simulink model "mixTest123"  (R2020a)
settings: Solver=VariableStepAuto  StartTime=0.0  StopTime=1000  FixedStep=0.05  RelTol=1e-3
InitFcn:
  | data_current
values from neighbouring files (symbols this model uses):
  a1 = rho * D^4 * alpha1    (= 0.000388302366464)    [data_current.m]    (also in main_init.m)
  a2 = -rho * D^3 * alpha2 * (1 - omega)    (= 0.0037030698432)    [data_current.m]    (also in main_init.m)
  ag = [Ax Ay Az]'    [init_modello.m]
  alpha1 = 0.0113    [data_current.m]    (also in main_init.m)
  alpha2 = -0.0091    [data_current.m]    (also in main_init.m)
  areaOfInterestCorner = [42.317744;10.915136; 0]    [init_controllo.m]    (also in missionA.m = [42.317744)
  bg = [Bx By Bz]'    [init_modello.m]
  cd_pitch = 0.7    [init_modello.m]
  cd_roll = 0.04    [init_modello.m]
  cd_x = 0.4    [init_modello.m]
  cd_y = 1    [init_modello.m]
  cd_yaw = 0.7    [init_modello.m]
  cd_z = 1    [init_modello.m]
  cg = [Cx Cy Cz]'    [init_modello.m]
  D = 0.076    [data_current.m]    (also in main_init.m)
  dead_zone_limit = 31.5    [data_current.m]    (also in main_init.m)
  dg = [Dx Dy Dz]'    [init_modello.m]
  eg = [Ex Ey Ez]'    [init_modello.m]
  fg = [Fx Fy Fz]'    [init_modello.m]
  g = 9.81    [init_modello.m]
  galleggiamento = 66.5386    [init_controllo.m]
  gg = [Gx Gy Gz]'    [init_modello.m]
  H0 = 0    [init_modello.m]
  init_position = [pointP(1),pointP(2),0.15,0,0,deg2rad(angle)]'    [appunti.m]    (also in init_modello.m = [pointP(1),pointP(2),0.15,0,0,deg2rad(alpha)]')
  init_velocity = [0 0 0 0 0 0]'    [init_modello.m]
  Ixx = 0.93304097392    [init_modello.m]
  Ixy = 0    [init_modello.m]
  Ixz = 0    [init_modello.m]
  Iyy = 25.58745481378    (= 25.5874548138)    [init_modello.m]
  Iyz = 0    [init_modello.m]
  Izz = 25.58745481378    (= 25.5874548138)    [init_modello.m]
  K_i_heave_div = 20    [init_controllo.m]
  K_i_heave_pos = 1    [init_controllo.m]
  K_i_heave_surf = 20    [init_controllo.m]
  K_i_heave_trans = 5    [init_controllo.m]
  K_i_heave_turn = 5    [init_controllo.m]
  K_i_pitch_div = 0    [init_controllo.m]
  K_i_pitch_pos = 0.1*0    (= 0)    [init_controllo.m]
  K_i_pitch_surf = 0    [init_controllo.m]
  K_i_pitch_trans = 0    [init_controllo.m]
  K_i_pitch_turn = 0    [init_controllo.m]
  K_i_roll_div = 0    [init_controllo.m]
  K_i_roll_pos = 0.1*0    (= 0)    [init_controllo.m]
  K_i_roll_surf = 1    [init_controllo.m]
  K_i_roll_trans = 0    [init_controllo.m]
  K_i_roll_turn = 0    [init_controllo.m]
  K_i_surge_div = 3    [init_controllo.m]
  K_i_surge_pos = 0.1679*30    (= 5.037)    [init_controllo.m]
  K_i_surge_surf = 3    [init_controllo.m]
  K_i_surge_trans = 0.1679*15    (= 2.5185)    [init_controllo.m]
  K_i_surge_turn = 0.1679*60    (= 10.074)    [init_controllo.m]
  K_i_sway_div = 6    [init_controllo.m]
  K_i_sway_pos = 5    [init_controllo.m]
  K_i_sway_surf = 3    [init_controllo.m]
  K_i_sway_trans = 2    [init_controllo.m]
  K_i_sway_turn = 50    [init_controllo.m]
  K_i_yaw_div = 0    [init_controllo.m]
  K_i_yaw_pos = 1    [init_controllo.m]
  K_i_yaw_surf = 0    [init_controllo.m]
  K_i_yaw_trans = 20    [init_controllo.m]
  K_i_yaw_turn = 3    [init_controllo.m]
  K_p_heave_div = 200    [init_controllo.m]
  K_p_heave_pos = 320    [init_controllo.m]
  K_p_heave_surf = 200    [init_controllo.m]
  K_p_heave_trans = 170    [init_controllo.m]
  K_p_heave_turn = 170    [init_controllo.m]
  K_p_phi_div = 0.15    [init_controllo.m]
  K_p_phi_pos = 1*0.1    (= 0.1)    [init_controllo.m]
  K_p_phi_surf = 0.15    [init_controllo.m]
  K_p_phi_trans = 0.1    [init_controllo.m]
  K_p_phi_turn = 0.1    [init_controllo.m]
  K_p_pitch_div = 50    [init_controllo.m]
  K_p_pitch_pos = 25    [init_controllo.m]
  K_p_pitch_surf = 50    [init_controllo.m]
  K_p_pitch_trans = 25    [init_controllo.m]
  K_p_pitch_turn = 25    [init_controllo.m]
  K_p_psi_div = 0.3    [init_controllo.m]
  K_p_psi_pos = 0.25    [init_controllo.m]
  K_p_psi_surf = 0.3    [init_controllo.m]
  K_p_psi_trans = 0.2    [init_controllo.m]
  K_p_roll_div = 10    [init_controllo.m]
  K_p_roll_pos = 0.1*40    (= 4)    [init_controllo.m]
  K_p_roll_surf = 10    [init_controllo.m]
  K_p_roll_trans = 0.1*40    (= 4)    [init_controllo.m]
  K_p_roll_turn = 4    [init_controllo.m]
  K_p_surge_div = 80    [init_controllo.m]
  K_p_surge_pos = 13.7782*2.5    (= 34.4455)    [init_controllo.m]
  K_p_surge_surf = 80    [init_controllo.m]
  K_p_surge_trans = 20    [init_controllo.m]
  K_p_surge_turn = 150    [init_controllo.m]
  K_p_sway_div = 100    [init_controllo.m]
  K_p_sway_pos = 90    [init_controllo.m]
  K_p_sway_surf = 80    [init_controllo.m]
  K_p_sway_trans = 80    [init_controllo.m]
  K_p_sway_turn = 200    [init_controllo.m]
  K_p_th_div = 0.3    [init_controllo.m]
  K_p_th_pos = 0.1    [init_controllo.m]
  K_p_th_surf = 0.3    [init_controllo.m]
  K_p_th_trans = 0.1    [init_controllo.m]
  K_p_th_turn = 0.1    [init_controllo.m]
  K_p_x_div = 0.12    [init_controllo.m]
  K_p_x_pos = 0.12    [init_controllo.m]
  K_p_x_surf = 0.12    [init_controllo.m]
  K_p_y_div = 0.6    [init_controllo.m]
  K_p_y_pos = 0.34    [init_controllo.m]
  K_p_y_surf = 0.1    [init_controllo.m]
  K_p_y_trans = 0.3    [init_controllo.m]
  K_p_y_turn = 0.3    [init_controllo.m]
  K_p_yaw_div = 70    [init_controllo.m]
  K_p_yaw_pos = 20    [init_controllo.m]
  K_p_yaw_surf = 70    [init_controllo.m]
  K_p_yaw_trans = 160    [init_controllo.m]
  K_p_yaw_turn = 60    [init_controllo.m]
  K_p_z_div = 0.35    [init_controllo.m]
  K_p_z_pos = 0.2    [init_controllo.m]
  K_p_z_surf = 0.35    [init_controllo.m]
  K_p_z_trans = 0.10    (= 0.1)    [init_controllo.m]
  K_p_z_turn = 0.1    [init_controllo.m]
  Kadd = 0    [init_modello.m]
  m = 100    [init_modello.m]    (also in retta.m = p2-p1)
  ... (+29 more)
undefined symbols (not defined in the file or in its folder): DiscIntNeverNeededParam
libraries: simulink x4
(part 2 of 5)

== system mixTest123/controller/turning controller/yaw_controller ==
  enable : Inport
  references : Inport  Port=2
  "estimated measures " : Inport  Port=3
  Yaw PID controller : Subsystem
  N : Outport
  wires:
  enable/1 -> Yaw PID controller/1(enable)
  "estimated measures "/1 -> Yaw PID controller/3(est_meas)
  references/1 -> Yaw PID controller/2(ref)
  Yaw PID controller/1(N) -> N/1  "N_pid"

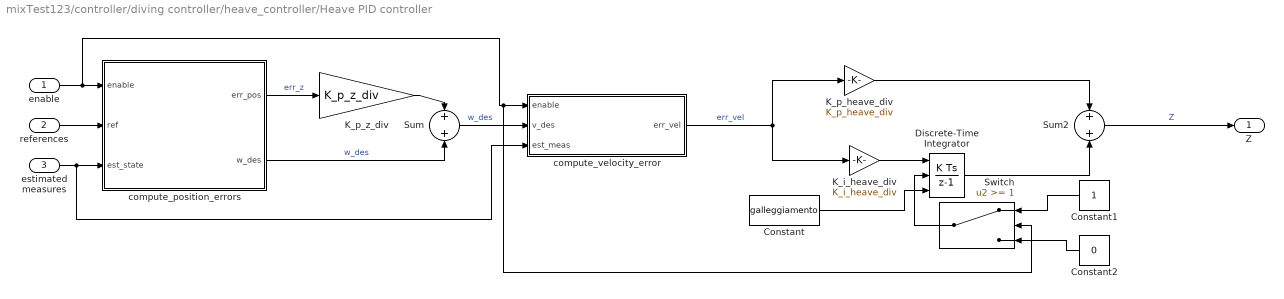
== system mixTest123/controller/diving controller/heave_controller/Heave PID controller ==
  enable : Inport
  references : Inport  Port=2
  "estimated measures " : Inport  Port=3
  Constant : Constant  Value=galleggiamento
  Constant1 : Constant
  Constant2 : Constant  Value=0
  Discrete-Time Integrator : DiscreteIntegrator  ExternalReset=falling  InitialConditionSource=external  SampleTime=0.1  ICPrevOutput=DiscIntNeverNeededParam  ICPrevScaledInput=DiscIntNeverNeededParam
  K_i_heave_div : Gain  Gain=K_i_heave_div
  K_p_heave_div : Gain  Gain=K_p_heave_div
  K_p_z_div : Gain  Gain=K_p_z_div
  Sum : Sum
  Sum2 : Sum
  Switch : Switch  Threshold=1
  compute_position_errors : MATLAB Function  TreatAsAtomicUnit=on
  compute_velocity_error : MATLAB Function  TreatAsAtomicUnit=on
  Z : Outport
  wires:
  "estimated measures "/1 -> compute_velocity_error/3(est_meas), compute_position_errors/3(est_state)
  K_p_z_div/1 -> Sum/1
  compute_position_errors/1(err_pos) -> K_p_z_div/1  "err_z"
  references/1 -> compute_position_errors/2(ref)
  Sum/1 -> compute_velocity_error/2(v_des)  "w_des"
  compute_position_errors/2(w_des) -> Sum/2  "w_des"
  K_p_heave_div/1 -> Sum2/1
  K_i_heave_div/1 -> Discrete-Time Integrator/1
  compute_velocity_error/1(err_vel) -> K_i_heave_div/1, K_p_heave_div/1  "err_vel"
  Sum2/1 -> Z/1  "Z"
  Discrete-Time Integrator/1 -> Sum2/2
  Constant/1 -> Discrete-Time Integrator/3
  Switch/1 -> Discrete-Time Integrator/2
  enable/1 -> Switch/2, compute_velocity_error/1(enable), compute_position_errors/1(enable)
  Constant2/1 -> Switch/3
  Constant1/1 -> Switch/1

== system mixTest123/controller/diving controller/pitch_controller/Pitch PID controller ==
  enable : Inport
  references : Inport  Port=2
  "estimated measures " : Inport  Port=3
  Constant : Constant
  Constant1 : Constant  Value=0
  Discrete-Time Integrator : DiscreteIntegrator  ExternalReset=falling  SampleTime=0.1  ICPrevOutput=DiscIntNeverNeededParam  ICPrevScaledInput=DiscIntNeverNeededParam
  K_i_pitch_div : Gain  Gain=K_i_pitch_div
  K_p_pitch_div : Gain  Gain=K_p_pitch_div
  K_p_th_div : Gain  Gain=K_p_th_div
  Sum2 : Sum
  Switch : Switch  Threshold=1
  compute_orientation_errors : MATLAB Function  TreatAsAtomicUnit=on
  compute_velocity_error : MATLAB Function  TreatAsAtomicUnit=on
  tau_pitch : Outport
  wires:
  references/1 -> compute_orientation_errors/2(ref)
  K_p_th_div/1 -> compute_velocity_error/2(v_des)
  "estimated measures "/1 -> compute_velocity_error/3(est_meas), compute_orientation_errors/3(est_state)
  compute_orientation_errors/1(err_orient) -> K_p_th_div/1  "err_orient"
  K_p_pitch_div/1 -> Sum2/1
  Sum2/1 -> tau_pitch/1  "tau_pitch"
  K_i_pitch_div/1 -> Discrete-Time Integrator/1
  Discrete-Time Integrator/1 -> Sum2/2
  compute_velocity_error/1(err_vel) -> K_i_pitch_div/1, K_p_pitch_div/1  "err_vel"
  Switch/1 -> Discrete-Time Integrator/2
  enable/1 -> Switch/2, compute_velocity_error/1(enable), compute_orientation_errors/1(enable)
  Constant1/1 -> Switch/3
  Constant/1 -> Switch/1

== system mixTest123/controller/diving controller/roll_controller/Roll PID controller ==
  enable : Inport
  references : Inport  Port=2
  "estimated measures " : Inport  Port=3
  Constant : Constant
  Constant1 : Constant  Value=0
  Discrete-Time Integrator : DiscreteIntegrator  ExternalReset=falling  SampleTime=0.1  ICPrevOutput=DiscIntNeverNeededParam  ICPrevScaledInput=DiscIntNeverNeededParam
  K_i_roll_div : Gain  Gain=K_i_roll_div
  K_p_phi_div : Gain  Gain=K_p_phi_div
  K_p_roll_div : Gain  Gain=K_p_roll_div
  Sum2 : Sum
  Switch : Switch  Threshold=1
  compute_orientation_errors : MATLAB Function  TreatAsAtomicUnit=on
  compute_velocity_error : MATLAB Function  TreatAsAtomicUnit=on
  tau_roll : Outport
  wires:
  "estimated measures "/1 -> compute_velocity_error/3(est_meas), compute_orientation_errors/3(est_state)
  K_p_phi_div/1 -> compute_velocity_error/2(v_des)
  compute_orientation_errors/1(err_orient) -> K_p_phi_div/1  "err_orient"
  references/1 -> compute_orientation_errors/2(ref)
  K_p_roll_div/1 -> Sum2/1
  Sum2/1 -> tau_roll/1  "tau_roll"
  K_i_roll_div/1 -> Discrete-Time Integrator/1
  Discrete-Time Integrator/1 -> Sum2/2
  compute_velocity_error/1(err_vel) -> K_i_roll_div/1, K_p_roll_div/1  "err_vel"
  Switch/1 -> Discrete-Time Integrator/2
  enable/1 -> Switch/2, compute_velocity_error/1(enable), compute_orientation_errors/1(enable)
  Constant1/1 -> Switch/3
  Constant/1 -> Switch/1

== system mixTest123/controller/diving controller/surge_controller/Surge PID controller ==
  enable : Inport
  references : Inport  Port=2
  "estimated measures " : Inport  Port=3
  Constant : Constant
  Constant1 : Constant  Value=0
  Discrete-Time Integrator : DiscreteIntegrator  ExternalReset=falling  SampleTime=0.1  ICPrevOutput=DiscIntNeverNeededParam  ICPrevScaledInput=DiscIntNeverNeededParam
  K_i_surge_div : Gain  Gain=K_i_surge_div
  K_p_surge_div : Gain  Gain=K_p_surge_div
  K_p_x_div : Gain  Gain=K_p_x_div
  Sum2 : Sum
  Switch : Switch  Threshold=1
  compute_position_errors : MATLAB Function  TreatAsAtomicUnit=on
  compute_velocity_error : MATLAB Function  TreatAsAtomicUnit=on
  X : Outport
  wires:
  references/1 -> compute_position_errors/2(ref)
  compute_position_errors/1(err_pos) -> K_p_x_div/1  "err_x"
  "estimated measures "/1 -> compute_velocity_error/3(est_meas), compute_position_errors/3(est_state)
  K_p_x_div/1 -> compute_velocity_error/2(v_des)
  Sum2/1 -> X/1  "X"
  K_p_surge_div/1 -> Sum2/1
  Discrete-Time Integrator/1 -> Sum2/2
  K_i_surge_div/1 -> Discrete-Time Integrator/1
  compute_velocity_error/1(err_vel) -> K_i_surge_div/1, K_p_surge_div/1  "err_vel"
  Switch/1 -> Discrete-Time Integrator/2
  enable/1 -> Switch/2, compute_velocity_error/1(enable), compute_position_errors/1(enable)
  Constant1/1 -> Switch/3
  Constant/1 -> Switch/1

== system mixTest123/controller/diving controller/sway_controller/Sway PID controller ==
  enable : Inport
  references : Inport  Port=2
  "estimated measures " : Inport  Port=3
  Constant : Constant
  Constant1 : Constant  Value=0
  Discrete-Time Integrator : DiscreteIntegrator  ExternalReset=falling  SampleTime=0.1  ICPrevOutput=DiscIntNeverNeededParam  ICPrevScaledInput=DiscIntNeverNeededParam
  K_i_sway_div : Gain  Gain=K_i_sway_div
  K_p_sway_div : Gain  Gain=K_p_sway_div
  K_p_y_div : Gain  Gain=K_p_y_div
  Sum2 : Sum
  Switch : Switch  Threshold=1
  compute_position_errors : MATLAB Function  TreatAsAtomicUnit=on
  compute_velocity_error : MATLAB Function  TreatAsAtomicUnit=on
  Y : Outport
  wires:
  references/1 -> compute_position_errors/2(ref)
  compute_position_errors/1(err_pos) -> K_p_y_div/1  "err_y"
  K_p_y_div/1 -> compute_velocity_error/2(v_des)  "v_des_sway"
  "estimated measures "/1 -> compute_velocity_error/3(est_meas), compute_position_errors/3(est_state)
  K_p_sway_div/1 -> Sum2/1
  Sum2/1 -> Y/1  "Y"
  K_i_sway_div/1 -> Discrete-Time Integrator/1
  Discrete-Time Integrator/1 -> Sum2/2
  compute_velocity_error/1(err_vel) -> K_i_sway_div/1, K_p_sway_div/1  "err_vel"
  Switch/1 -> Discrete-Time Integrator/2
  enable/1 -> Switch/2, compute_velocity_error/1(enable), compute_position_errors/1(enable)
  Constant1/1 -> Switch/3
  Constant/1 -> Switch/1

== system mixTest123/controller/diving controller/yaw_controller/Yaw PID controller ==
  enable : Inport
  references : Inport  Port=2
  "estimated measures " : Inport  Port=3
  Constant : Constant
  Constant1 : Constant  Value=0
  Discrete-Time Integrator : DiscreteIntegrator  ExternalReset=falling  SampleTime=0.1  ICPrevOutput=DiscIntNeverNeededParam  ICPrevScaledInput=DiscIntNeverNeededParam
  K_i_yaw_div : Gain  Gain=K_i_yaw_div
  K_p_psi_div : Gain  Gain=K_p_psi_div
  K_p_yaw_div : Gain  Gain=K_p_yaw_div
  Sum2 : Sum
  Switch : Switch  Threshold=1
  compute_orientation_errors : MATLAB Function  TreatAsAtomicUnit=on
  compute_velocity_error : MATLAB Function  TreatAsAtomicUnit=on
  tau_yaw : Outport
  wires:
  references/1 -> compute_orientation_errors/2(ref)
  "estimated measures "/1 -> compute_velocity_error/3(est_meas), compute_orientation_errors/3(est_state)
  compute_orientation_errors/1(err_orient) -> K_p_psi_div/1  "err_orient"
  K_p_psi_div/1 -> compute_velocity_error/2(v_des)
  K_p_yaw_div/1 -> Sum2/1
  Sum2/1 -> tau_yaw/1  "tau_yaw"
  K_i_yaw_div/1 -> Discrete-Time Integrator/1
  Discrete-Time Integrator/1 -> Sum2/2
  compute_velocity_error/1(err_vel) -> K_i_yaw_div/1, K_p_yaw_div/1  "err_vel"
  Switch/1 -> Discrete-Time Integrator/2
  enable/1 -> compute_velocity_error/1(enable), Switch/2, compute_orientation_errors/1(enable)
  Constant1/1 -> Switch/3
  Constant/1 -> Switch/1

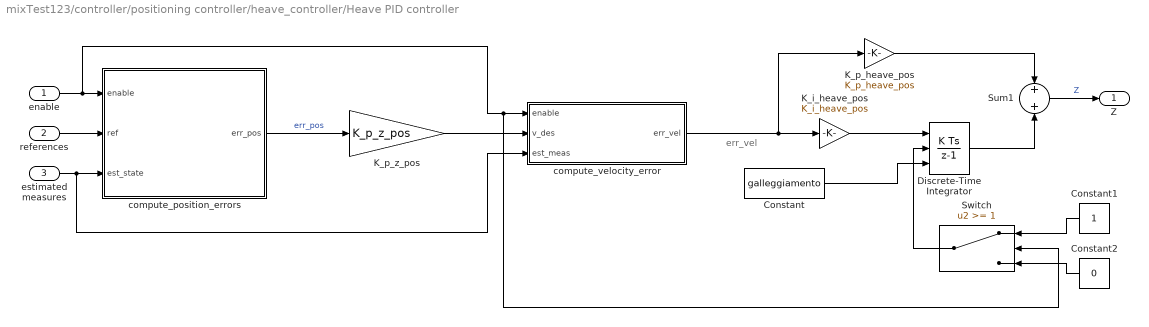
== system mixTest123/controller/positioning controller/heave_controller/Heave PID controller ==
  note: err_vel
  enable : Inport
  references : Inport  Port=2
  "estimated measures " : Inport  Port=3
  Constant : Constant  Value=galleggiamento
  Constant1 : Constant
  Constant2 : Constant  Value=0
  Discrete-Time Integrator : DiscreteIntegrator  ExternalReset=falling  InitialConditionSource=external  SampleTime=0.1  ICPrevOutput=DiscIntNeverNeededParam  ICPrevScaledInput=DiscIntNeverNeededParam
  K_i_heave_pos : Gain  Gain=K_i_heave_pos
  K_p_heave_pos : Gain  Gain=K_p_heave_pos
  K_p_z_pos : Gain  Gain=K_p_z_pos
  Sum1 : Sum
  Switch : Switch  Threshold=1
  compute_position_errors : MATLAB Function  TreatAsAtomicUnit=on
  compute_velocity_error : MATLAB Function  TreatAsAtomicUnit=on
  Z : Outport
  wires:
  "estimated measures "/1 -> compute_velocity_error/3(est_meas), compute_position_errors/3(est_state)
  K_p_z_pos/1 -> compute_velocity_error/2(v_des)
  compute_position_errors/1(err_pos) -> K_p_z_pos/1  "err_pos"
  references/1 -> compute_position_errors/2(ref)
  K_i_heave_pos/1 -> Discrete-Time Integrator/1
  compute_velocity_error/1(err_vel) -> K_i_heave_pos/1, K_p_heave_pos/1
  K_p_heave_pos/1 -> Sum1/1
  Discrete-Time Integrator/1 -> Sum1/2
  Sum1/1 -> Z/1  "Z"
  Constant/1 -> Discrete-Time Integrator/3
  Switch/1 -> Discrete-Time Integrator/2
  enable/1 -> compute_velocity_error/1(enable), Switch/2, compute_position_errors/1(enable)
  Constant2/1 -> Switch/3
  Constant1/1 -> Switch/1

== system mixTest123/controller/positioning controller/pitch_controller/Pitch PID controller ==
  enable : Inport
  references : Inport  Port=2
  "estimated measures " : Inport  Port=3
  Constant : Constant
  Constant1 : Constant  Value=0
  Discrete-Time Integrator : DiscreteIntegrator  ExternalReset=falling  SampleTime=0.1  ICPrevOutput=DiscIntNeverNeededParam  ICPrevScaledInput=DiscIntNeverNeededParam
  K_i_pitch_pos : Gain  Gain=K_i_pitch_pos
  K_p_pitch_pos : Gain  Gain=K_p_pitch_pos
  K_p_th_pos : Gain  Gain=K_p_th_pos
  Sum1 : Sum
  Switch : Switch  Threshold=1
  compute_orientation_errors : MATLAB Function  TreatAsAtomicUnit=on
  compute_velocity_error : MATLAB Function  TreatAsAtomicUnit=on
  tau_pitch : Outport
  wires:
  references/1 -> compute_orientation_errors/2(ref)
  K_p_th_pos/1 -> compute_velocity_error/2(v_des)
  Sum1/1 -> tau_pitch/1  "tau_pitch"
  "estimated measures "/1 -> compute_velocity_error/3(est_meas), compute_orientation_errors/3(est_state)
  compute_orientation_errors/1(err_orient) -> K_p_th_pos/1  "err_orient"
  K_i_pitch_pos/1 -> Discrete-Time Integrator/1
  compute_velocity_error/1(err_vel) -> K_i_pitch_pos/1, K_p_pitch_pos/1  "err_vel"
  Discrete-Time Integrator/1 -> Sum1/2
  K_p_pitch_pos/1 -> Sum1/1
  Switch/1 -> Discrete-Time Integrator/2
  enable/1 -> Switch/2, compute_velocity_error/1(enable), compute_orientation_errors/1(enable)
  Constant1/1 -> Switch/3
  Constant/1 -> Switch/1

== system mixTest123/controller/positioning controller/roll_controller/Roll PID controller ==
  note: err_vel
  enable : Inport
  references : Inport  Port=2
  "estimated measures " : Inport  Port=3
  Constant : Constant
  Constant1 : Constant  Value=0
  Discrete-Time Integrator : DiscreteIntegrator  ExternalReset=falling  SampleTime=0.1  ICPrevOutput=DiscIntNeverNeededParam  ICPrevScaledInput=DiscIntNeverNeededParam
  K_i_roll_pos : Gain  Gain=K_i_roll_pos
  K_p_phi_pos : Gain  Gain=K_p_phi_pos
  K_p_roll_pos : Gain  Gain=K_p_roll_pos
  Sum1 : Sum
  Switch : Switch  Threshold=1
  compute_orientation_errors : MATLAB Function  TreatAsAtomicUnit=on
  compute_velocity_error : MATLAB Function  TreatAsAtomicUnit=on
  tau_roll : Outport
  wires:
  "estimated measures "/1 -> compute_velocity_error/3(est_meas), compute_orientation_errors/3(est_state)
  Sum1/1 -> tau_roll/1  "tau_roll"
  K_p_phi_pos/1 -> compute_velocity_error/2(v_des)  "v_des"
  compute_orientation_errors/1(err_orient) -> K_p_phi_pos/1  "err_orient"
  references/1 -> compute_orientation_errors/2(ref)
  K_i_roll_pos/1 -> Discrete-Time Integrator/1
  compute_velocity_error/1(err_vel) -> K_i_roll_pos/1, K_p_roll_pos/1
  Discrete-Time Integrator/1 -> Sum1/2
  K_p_roll_pos/1 -> Sum1/1
  Switch/1 -> Discrete-Time Integrator/2
  enable/1 -> Switch/2, compute_velocity_error/1(enable), compute_orientation_errors/1(enable)
  Constant1/1 -> Switch/3
  Constant/1 -> Switch/1

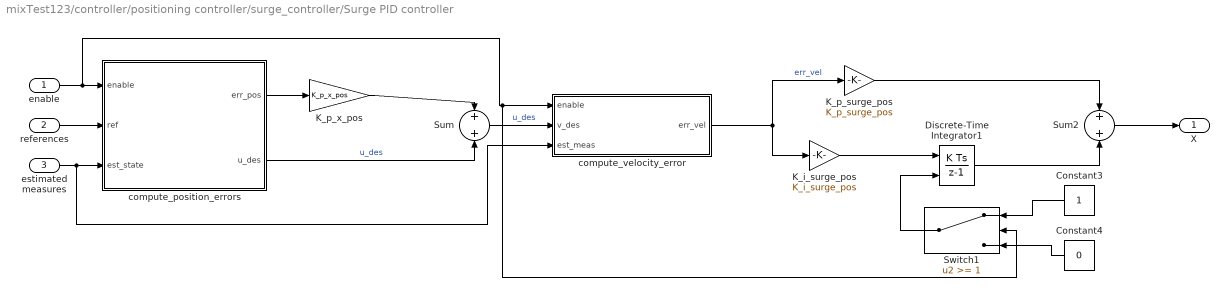
== system mixTest123/controller/positioning controller/surge_controller/Surge PID controller ==
  enable : Inport
  references : Inport  Port=2
  "estimated measures " : Inport  Port=3
  Constant3 : Constant
  Constant4 : Constant  Value=0
  Discrete-Time Integrator1 : DiscreteIntegrator  ExternalReset=falling  SampleTime=0.1  ICPrevOutput=DiscIntNeverNeededParam  ICPrevScaledInput=DiscIntNeverNeededParam
  K_i_surge_pos : Gain  Gain=K_i_surge_pos
  K_p_surge_pos : Gain  Gain=K_p_surge_pos
  K_p_x_pos : Gain  Gain=K_p_x_pos
  Sum : Sum
  Sum2 : Sum
  Switch1 : Switch  Threshold=1
  compute_position_errors : MATLAB Function  TreatAsAtomicUnit=on
  compute_velocity_error : MATLAB Function  TreatAsAtomicUnit=on
  X : Outport
  wires:
  Constant3/1 -> Switch1/1
  Constant4/1 -> Switch1/3
  compute_position_errors/1(err_pos) -> K_p_x_pos/1
  K_i_surge_pos/1 -> Discrete-Time Integrator1/1
  Switch1/1 -> Discrete-Time Integrator1/2
  compute_position_errors/2(u_des) -> Sum/2  "u_des"
  Sum/1 -> compute_velocity_error/2(v_des)  "u_des"
  Sum2/1 -> X/1
  K_p_surge_pos/1 -> Sum2/1
  compute_velocity_error/1(err_vel) -> K_i_surge_pos/1, K_p_surge_pos/1  "err_vel"
  "estimated measures "/1 -> compute_velocity_error/3(est_meas), compute_position_errors/3(est_state)
  references/1 -> compute_position_errors/2(ref)
  K_p_x_pos/1 -> Sum/1
  enable/1 -> Switch1/2, compute_velocity_error/1(enable), compute_position_errors/1(enable)
  Discrete-Time Integrator1/1 -> Sum2/2

== system mixTest123/controller/positioning controller/sway_controller/Sway PID controller ==
  enable : Inport
  references : Inport  Port=2
  "estimated measures " : Inport  Port=3
  Constant : Constant
  Constant1 : Constant  Value=0
  Discrete-Time Integrator : DiscreteIntegrator  ExternalReset=falling  SampleTime=0.1  ICPrevOutput=DiscIntNeverNeededParam  ICPrevScaledInput=DiscIntNeverNeededParam
  K_i_sway_pos : Gain  Gain=K_i_sway_pos
  K_p_sway_pos : Gain  Gain=K_p_sway_pos
  K_p_y_pos : Gain  Gain=K_p_y_pos
  Sum1 : Sum
  Switch : Switch  Threshold=1
  compute_position_errors : MATLAB Function  TreatAsAtomicUnit=on
  compute_velocity_error : MATLAB Function  TreatAsAtomicUnit=on
  Y : Outport
  wires:
  references/1 -> compute_position_errors/2(ref)
  K_p_y_pos/1 -> compute_velocity_error/2(v_des)
  "estimated measures "/1 -> compute_velocity_error/3(est_meas), compute_position_errors/3(est_state)
  K_i_sway_pos/1 -> Discrete-Time Integrator/1
  compute_velocity_error/1(err_vel) -> K_i_sway_pos/1, K_p_sway_pos/1  "err_vel"
  Discrete-Time Integrator/1 -> Sum1/2
  K_p_sway_pos/1 -> Sum1/1
  Sum1/1 -> Y/1  "Y"
  compute_position_errors/1(err_pos) -> K_p_y_pos/1  "err_y"
  Switch/1 -> Discrete-Time Integrator/2
  enable/1 -> Switch/2, compute_velocity_error/1(enable), compute_position_errors/1(enable)
  Constant1/1 -> Switch/3
  Constant/1 -> Switch/1

== system mixTest123/controller/positioning controller/yaw_controller/Yaw PID controller ==
  enable : Inport
  references : Inport  Port=2
  "estimated measures " : Inport  Port=3
  Constant : Constant
  Constant1 : Constant  Value=0
  Discrete-Time Integrator : DiscreteIntegrator  ExternalReset=falling  SampleTime=0.1  ICPrevOutput=DiscIntNeverNeededParam  ICPrevScaledInput=DiscIntNeverNeededParam
  K_i_yaw_pos : Gain  Gain=K_i_yaw_pos
  K_p_psi_pos : Gain  Gain=K_p_psi_pos
  K_p_yaw_pos : Gain  Gain=K_p_yaw_pos
  Sum1 : Sum
  Switch : Switch  Threshold=1
  compute_orientation_errors : MATLAB Function  TreatAsAtomicUnit=on
  compute_velocity_error : MATLAB Function  TreatAsAtomicUnit=on
  tau_yaw : Outport
  wires:
  references/1 -> compute_orientation_errors/2(ref)
  Sum1/1 -> tau_yaw/1  "tau_yaw"
  "estimated measures "/1 -> compute_velocity_error/3(est_meas), compute_orientation_errors/3(est_state)
  compute_orientation_errors/1(err_orient) -> K_p_psi_pos/1  "err_orient"
  K_p_psi_pos/1 -> compute_velocity_error/2(v_des)
  K_i_yaw_pos/1 -> Discrete-Time Integrator/1
  compute_velocity_error/1(err_vel) -> K_i_yaw_pos/1, K_p_yaw_pos/1  "err_vel"
  Discrete-Time Integrator/1 -> Sum1/2
  K_p_yaw_pos/1 -> Sum1/1
  Switch/1 -> Discrete-Time Integrator/2
  enable/1 -> Switch/2, compute_velocity_error/1(enable), compute_orientation_errors/1(enable)
  Constant1/1 -> Switch/3
  Constant/1 -> Switch/1

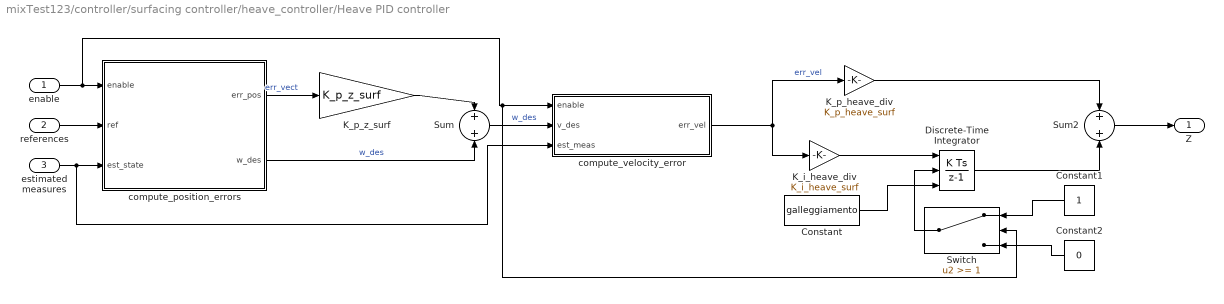
== system mixTest123/controller/surfacing controller/heave_controller/Heave PID controller ==
  enable : Inport
  references : Inport  Port=2
  "estimated measures " : Inport  Port=3
  Constant : Constant  Value=galleggiamento
  Constant1 : Constant
  Constant2 : Constant  Value=0
  Discrete-Time Integrator : DiscreteIntegrator  ExternalReset=falling  InitialConditionSource=external  SampleTime=0.1  ICPrevOutput=DiscIntNeverNeededParam  ICPrevScaledInput=DiscIntNeverNeededParam
  K_i_heave_div : Gain  Gain=K_i_heave_surf
  K_p_heave_div : Gain  Gain=K_p_heave_surf
  K_p_z_surf : Gain  Gain=K_p_z_surf
  Sum : Sum
  Sum2 : Sum
  Switch : Switch  Threshold=1
  compute_position_errors : MATLAB Function  TreatAsAtomicUnit=on
  compute_velocity_error : MATLAB Function  TreatAsAtomicUnit=on
  Z : Outport
  wires:
  K_i_heave_div/1 -> Discrete-Time Integrator/1
  K_p_heave_div/1 -> Sum2/1
  references/1 -> compute_position_errors/2(ref)
  "estimated measures "/1 -> compute_velocity_error/3(est_meas), compute_position_errors/3(est_state)
  Sum/1 -> compute_velocity_error/2(v_des)  "w_des"
  compute_position_errors/1(err_pos) -> K_p_z_surf/1  "err_vect"
  compute_position_errors/2(w_des) -> Sum/2  "w_des"
  Sum2/1 -> Z/1
  K_p_z_surf/1 -> Sum/1
  compute_velocity_error/1(err_vel) -> K_i_heave_div/1, K_p_heave_div/1  "err_vel"
  Discrete-Time Integrator/1 -> Sum2/2
  Constant/1 -> Discrete-Time Integrator/3
  Switch/1 -> Discrete-Time Integrator/2
  enable/1 -> Switch/2, compute_velocity_error/1(enable), compute_position_errors/1(enable)
  Constant2/1 -> Switch/3
  Constant1/1 -> Switch/1

== system mixTest123/controller/surfacing controller/pitch_controller/Pitch PID controller ==
  enable : Inport
  references : Inport  Port=2
  "estimated measures " : Inport  Port=3
  Constant : Constant
  Constant1 : Constant  Value=0
  Discrete-Time Integrator : DiscreteIntegrator  ExternalReset=falling  SampleTime=0.1  ICPrevOutput=DiscIntNeverNeededParam  ICPrevScaledInput=DiscIntNeverNeededParam
  K_i_pitch_surf : Gain  Gain=K_i_pitch_surf
  K_p_pitch_surf : Gain  Gain=K_p_pitch_surf
  K_p_th_surf : Gain  Gain=K_p_th_surf
  Sum2 : Sum
  Switch : Switch  Threshold=1
  compute_orientation_errors : MATLAB Function  TreatAsAtomicUnit=on
  compute_velocity_error : MATLAB Function  TreatAsAtomicUnit=on
  M : Outport
  wires:
  references/1 -> compute_orientation_errors/2(ref)
  K_p_th_surf/1 -> compute_velocity_error/2(v_des)
  "estimated measures "/1 -> compute_velocity_error/3(est_meas), compute_orientation_errors/3(est_state)
  compute_orientation_errors/1(err_orient) -> K_p_th_surf/1  "err_orient"
  Sum2/1 -> M/1
  Discrete-Time Integrator/1 -> Sum2/2
  K_i_pitch_surf/1 -> Discrete-Time Integrator/1
  K_p_pitch_surf/1 -> Sum2/1
  compute_velocity_error/1(err_vel) -> K_i_pitch_surf/1, K_p_pitch_surf/1  "err_vel"
  Switch/1 -> Discrete-Time Integrator/2
  enable/1 -> Switch/2, compute_velocity_error/1(enable), compute_orientation_errors/1(enable)
  Constant1/1 -> Switch/3
  Constant/1 -> Switch/1

== system mixTest123/controller/surfacing controller/roll_controller/Roll PID controller ==
  enable : Inport
  references : Inport  Port=2
  "estimated measures " : Inport  Port=3
  Constant : Constant
  Constant1 : Constant  Value=0
  Discrete-Time Integrator : DiscreteIntegrator  ExternalReset=falling  SampleTime=0.1  ICPrevOutput=DiscIntNeverNeededParam  ICPrevScaledInput=DiscIntNeverNeededParam
  K_i_roll_surf : Gain  Gain=K_i_roll_surf
  K_p_phi_surf : Gain  Gain=K_p_phi_surf
  K_p_roll_surf : Gain  Gain=K_p_roll_surf
  Sum2 : Sum
  Switch : Switch  Threshold=1
  compute_orientation_errors : MATLAB Function  TreatAsAtomicUnit=on
  compute_velocity_error : MATLAB Function  TreatAsAtomicUnit=on
  K : Outport
  wires:
  "estimated measures "/1 -> compute_velocity_error/3(est_meas), compute_orientation_errors/3(est_state)
  K_p_phi_surf/1 -> compute_velocity_error/2(v_des)
  compute_orientation_errors/1(err_orient) -> K_p_phi_surf/1  "err_orient"
  references/1 -> compute_orientation_errors/2(ref)
  Sum2/1 -> K/1
  Discrete-Time Integrator/1 -> Sum2/2
  K_i_roll_surf/1 -> Discrete-Time Integrator/1
  K_p_roll_surf/1 -> Sum2/1
  compute_velocity_error/1(err_vel) -> K_i_roll_surf/1, K_p_roll_surf/1  "err_vel"
  Switch/1 -> Discrete-Time Integrator/2
  enable/1 -> Switch/2, compute_velocity_error/1(enable), compute_orientation_errors/1(enable)
  Constant1/1 -> Switch/3
  Constant/1 -> Switch/1

== system mixTest123/controller/surfacing controller/surge_controller/Surge PID controller ==
  enable : Inport
  references : Inport  Port=2
  "estimated measures " : Inport  Port=3
  Constant : Constant
  Constant1 : Constant  Value=0
  Discrete-Time Integrator : DiscreteIntegrator  ExternalReset=falling  SampleTime=0.1  ICPrevOutput=DiscIntNeverNeededParam  ICPrevScaledInput=DiscIntNeverNeededParam
  K_i_surge_surf : Gain  Gain=K_i_surge_surf
  K_p_surge_surf : Gain  Gain=K_p_surge_surf
  K_p_x_surf : Gain  Gain=K_p_x_surf
  Sum2 : Sum
  Switch : Switch  Threshold=1
  compute_position_errors : MATLAB Function  TreatAsAtomicUnit=on
  compute_velocity_error : MATLAB Function  TreatAsAtomicUnit=on
  X : Outport
  wires:
  references/1 -> compute_position_errors/2(ref)
  compute_position_errors/1(err_pos) -> K_p_x_surf/1  "err_vect"
  K_p_x_surf/1 -> compute_velocity_error/2(v_des)
  "estimated measures "/1 -> compute_velocity_error/3(est_meas), compute_position_errors/3(est_state)
  K_i_surge_surf/1 -> Discrete-Time Integrator/1
  K_p_surge_surf/1 -> Sum2/1
  Sum2/1 -> X/1
  compute_velocity_error/1(err_vel) -> K_i_surge_surf/1, K_p_surge_surf/1  "err_vel"
  Discrete-Time Integrator/1 -> Sum2/2
  Switch/1 -> Discrete-Time Integrator/2
  enable/1 -> Switch/2, compute_velocity_error/1(enable), compute_position_errors/1(enable)
  Constant1/1 -> Switch/3
  Constant/1 -> Switch/1

== system mixTest123/controller/surfacing controller/sway_controller/Sway PID controller ==
  enable : Inport
  references : Inport  Port=2
  "estimated measures " : Inport  Port=3
  Constant : Constant
  Constant1 : Constant  Value=0
  Discrete-Time Integrator : DiscreteIntegrator  ExternalReset=falling  SampleTime=0.1  ICPrevOutput=DiscIntNeverNeededParam  ICPrevScaledInput=DiscIntNeverNeededParam
  K_i_sway_surf : Gain  Gain=K_i_sway_surf
  K_p_sway_surf : Gain  Gain=K_p_sway_surf
  K_p_y_surf : Gain  Gain=K_p_y_surf
  Sum2 : Sum
  Switch : Switch  Threshold=1
  compute_position_errors : MATLAB Function  TreatAsAtomicUnit=on
  compute_velocity_error : MATLAB Function  TreatAsAtomicUnit=on
  Y : Outport
  wires:
  references/1 -> compute_position_errors/2(ref)
  compute_position_errors/1(err_pos) -> K_p_y_surf/1  "err_y"
  K_p_y_surf/1 -> compute_velocity_error/2(v_des)
  "estimated measures "/1 -> compute_velocity_error/3(est_meas), compute_position_errors/3(est_state)
  K_i_sway_surf/1 -> Discrete-Time Integrator/1
  K_p_sway_surf/1 -> Sum2/1
  Sum2/1 -> Y/1
  compute_velocity_error/1(err_vel) -> K_i_sway_surf/1, K_p_sway_surf/1  "err_vel"
  Discrete-Time Integrator/1 -> Sum2/2
  Switch/1 -> Discrete-Time Integrator/2
  enable/1 -> Switch/2, compute_velocity_error/1(enable), compute_position_errors/1(enable)
  Constant1/1 -> Switch/3
  Constant/1 -> Switch/1

== system mixTest123/controller/surfacing controller/yaw_controller/Yaw PID controller ==
  enable : Inport
  references : Inport  Port=2
  "estimated measures " : Inport  Port=3
  Constant : Constant
  Constant1 : Constant  Value=0
  Discrete-Time Integrator : DiscreteIntegrator  ExternalReset=falling  SampleTime=0.1  ICPrevOutput=DiscIntNeverNeededParam  ICPrevScaledInput=DiscIntNeverNeededParam
  K_i_yaw_surf : Gain  Gain=K_i_yaw_surf
  K_p_psi_surf : Gain  Gain=K_p_psi_surf
  K_p_yaw_surf : Gain  Gain=K_p_yaw_surf
  Sum2 : Sum
  Switch : Switch  Threshold=1
  compute_orientation_errors : MATLAB Function  TreatAsAtomicUnit=on
  compute_velocity_error : MATLAB Function  TreatAsAtomicUnit=on
  N : Outport
  wires:
  references/1 -> compute_orientation_errors/2(ref)
  "estimated measures "/1 -> compute_velocity_error/3(est_meas), compute_orientation_errors/3(est_state)
  compute_orientation_errors/1(err_orient) -> K_p_psi_surf/1  "err_orient"
  K_p_psi_surf/1 -> compute_velocity_error/2(v_des)
  Sum2/1 -> N/1
  Discrete-Time Integrator/1 -> Sum2/2
  K_i_yaw_surf/1 -> Discrete-Time Integrator/1
  K_p_yaw_surf/1 -> Sum2/1
  compute_velocity_error/1(err_vel) -> K_i_yaw_surf/1, K_p_yaw_surf/1  "err_vel"
  Switch/1 -> Discrete-Time Integrator/2
  enable/1 -> Switch/2, compute_velocity_error/1(enable), compute_orientation_errors/1(enable)
  Constant1/1 -> Switch/3
  Constant/1 -> Switch/1

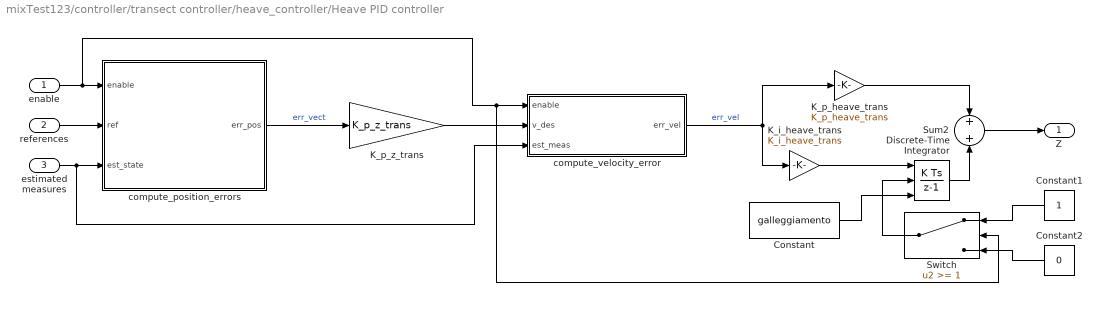
== system mixTest123/controller/transect controller/heave_controller/Heave PID controller ==
  enable : Inport
  references : Inport  Port=2
  "estimated measures " : Inport  Port=3
  Constant : Constant  Value=galleggiamento
  Constant1 : Constant
  Constant2 : Constant  Value=0
  Discrete-Time Integrator : DiscreteIntegrator  ExternalReset=falling  InitialConditionSource=external  SampleTime=0.1  ICPrevOutput=DiscIntNeverNeededParam  ICPrevScaledInput=DiscIntNeverNeededParam
  K_i_heave_trans : Gain  Gain=K_i_heave_trans
  K_p_heave_trans : Gain  Gain=K_p_heave_trans
  K_p_z_trans : Gain  Gain=K_p_z_trans
  Sum2 : Sum
  Switch : Switch  Threshold=1
  compute_position_errors : MATLAB Function  TreatAsAtomicUnit=on
  compute_velocity_error : MATLAB Function  TreatAsAtomicUnit=on
  Z : Outport
  wires:
  "estimated measures "/1 -> compute_velocity_error/3(est_meas), compute_position_errors/3(est_state)
  K_p_z_trans/1 -> compute_velocity_error/2(v_des)
  compute_position_errors/1(err_pos) -> K_p_z_trans/1  "err_vect"
  references/1 -> compute_position_errors/2(ref)
  Sum2/1 -> Z/1
  Discrete-Time Integrator/1 -> Sum2/2
  K_p_heave_trans/1 -> Sum2/1
  K_i_heave_trans/1 -> Discrete-Time Integrator/1
  compute_velocity_error/1(err_vel) -> K_i_heave_trans/1, K_p_heave_trans/1  "err_vel"
  Constant/1 -> Discrete-Time Integrator/3
  Switch/1 -> Discrete-Time Integrator/2
  enable/1 -> Switch/2, compute_velocity_error/1(enable), compute_position_errors/1(enable)
  Constant2/1 -> Switch/3
  Constant1/1 -> Switch/1

== system mixTest123/controller/transect controller/pitch_controller/Pitch PID controller ==
  enable : Inport
  references : Inport  Port=2
  "estimated measures " : Inport  Port=3
  Constant : Constant
  Constant1 : Constant  Value=0
  Discrete-Time Integrator : DiscreteIntegrator  ExternalReset=falling  SampleTime=0.1  ICPrevOutput=DiscIntNeverNeededParam  ICPrevScaledInput=DiscIntNeverNeededParam
  K_i_pitch_trans : Gain  Gain=K_i_pitch_trans
  K_p_pitch_trans : Gain  Gain=K_p_pitch_trans
  K_p_th_trans : Gain  Gain=K_p_th_trans
  Sum2 : Sum
  Switch : Switch  Threshold=1
  compute_orientation_errors : MATLAB Function  TreatAsAtomicUnit=on
  compute_velocity_error : MATLAB Function  TreatAsAtomicUnit=on
  M : Outport
  wires:
  references/1 -> compute_orientation_errors/2(ref)
  K_p_th_trans/1 -> compute_velocity_error/2(v_des)
  "estimated measures "/1 -> compute_velocity_error/3(est_meas), compute_orientation_errors/3(est_state)
  compute_orientation_errors/1(err_orient) -> K_p_th_trans/1  "err_orient"
  Sum2/1 -> M/1
  Discrete-Time Integrator/1 -> Sum2/2
  K_p_pitch_trans/1 -> Sum2/1
  K_i_pitch_trans/1 -> Discrete-Time Integrator/1
  compute_velocity_error/1(err_vel) -> K_i_pitch_trans/1, K_p_pitch_trans/1  "err_vel"
  Switch/1 -> Discrete-Time Integrator/2
  enable/1 -> Switch/2, compute_velocity_error/1(enable), compute_orientation_errors/1(enable)
  Constant1/1 -> Switch/3
  Constant/1 -> Switch/1

== system mixTest123/controller/transect controller/roll_controller/Roll PID controller ==
  enable : Inport
  references : Inport  Port=2
  "estimated measures " : Inport  Port=3
  Constant : Constant
  Constant1 : Constant  Value=0
  Discrete-Time Integrator : DiscreteIntegrator  ExternalReset=falling  SampleTime=0.1  ICPrevOutput=DiscIntNeverNeededParam  ICPrevScaledInput=DiscIntNeverNeededParam
  K_i_roll_trans : Gain  Gain=K_i_roll_trans
  K_p_phi_trans : Gain  Gain=K_p_phi_trans
  K_p_roll_trans : Gain  Gain=K_p_roll_trans
  Sum2 : Sum
  Switch : Switch  Threshold=1
  compute_orientation_errors : MATLAB Function  TreatAsAtomicUnit=on
  compute_velocity_error : MATLAB Function  TreatAsAtomicUnit=on
  tau_roll : Outport
  wires:
  "estimated measures "/1 -> compute_velocity_error/3(est_meas), compute_orientation_errors/3(est_state)
  K_p_phi_trans/1 -> compute_velocity_error/2(v_des)
  compute_orientation_errors/1(err_orient) -> K_p_phi_trans/1  "err_orient"
  references/1 -> compute_orientation_errors/2(ref)
  Sum2/1 -> tau_roll/1
  Discrete-Time Integrator/1 -> Sum2/2
  K_p_roll_trans/1 -> Sum2/1
  K_i_roll_trans/1 -> Discrete-Time Integrator/1
  compute_velocity_error/1(err_vel) -> K_p_roll_trans/1, K_i_roll_trans/1  "err_vel"
  Switch/1 -> Discrete-Time Integrator/2
  Constant1/1 -> Switch/3
  Constant/1 -> Switch/1
  enable/1 -> Switch/2, compute_velocity_error/1(enable), compute_orientation_errors/1(enable)

== system mixTest123/controller/transect controller/surge_controller/Surge PID controller ==
  enable : Inport
  ref : Inport  Port=2
  est_meas : Inport  Port=3
  " compute_velocity_error" : MATLAB Function  TreatAsAtomicUnit=on
  Constant : Constant
  Constant1 : Constant  Value=0
  Discrete-Time Integrator : DiscreteIntegrator  ExternalReset=falling  SampleTime=0.1  ICPrevOutput=DiscIntNeverNeededParam  ICPrevScaledInput=DiscIntNeverNeededParam
  K_i_surge_trans : Gain  Gain=K_i_surge_trans
  K_p_surge_trans : Gain  Gain=K_p_surge_trans
  Scope : Scope
  Sum2 : Sum
  Switch : Switch  Threshold=1
  X : Outport
  wires:
  est_meas/1 -> " compute_velocity_error"/3(est_meas)
  ref/1 -> " compute_velocity_error"/2(ref)
  " compute_velocity_error"/1(err_vel) -> K_i_surge_trans/1, K_p_surge_trans/1  "err_vel"
  K_p_surge_trans/1 -> Sum2/1
  Sum2/1 -> Scope/1, X/1  "X"
  K_i_surge_trans/1 -> Discrete-Time Integrator/1
  Discrete-Time Integrator/1 -> Sum2/2
  Switch/1 -> Discrete-Time Integrator/2
  enable/1 -> Switch/2, " compute_velocity_error"/1(enable)
  Constant1/1 -> Switch/3
  Constant/1 -> Switch/1

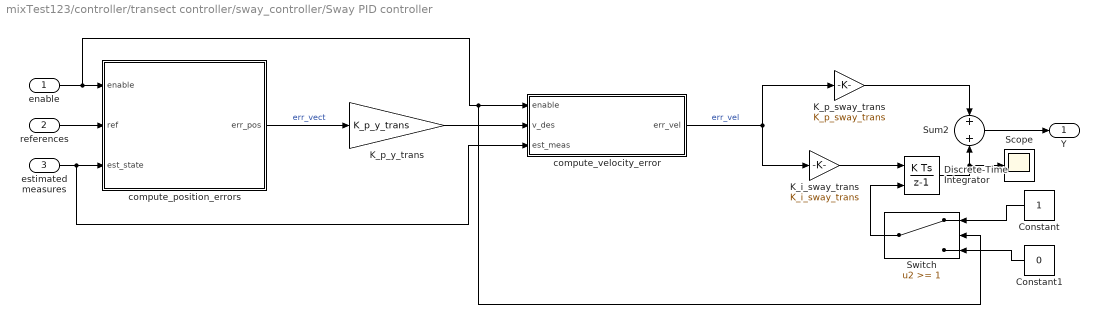
== system mixTest123/controller/transect controller/sway_controller/Sway PID controller ==
  enable : Inport
  references : Inport  Port=2
  "estimated measures " : Inport  Port=3
  Constant : Constant
  Constant1 : Constant  Value=0
  Discrete-Time Integrator : DiscreteIntegrator  ExternalReset=falling  SampleTime=0.1  LimitOutput=on  ICPrevOutput=DiscIntNeverNeededParam  ICPrevScaledInput=DiscIntNeverNeededParam
  K_i_sway_trans : Gain  Gain=K_i_sway_trans
  K_p_sway_trans : Gain  Gain=K_p_sway_trans
  K_p_y_trans : Gain  Gain=K_p_y_trans
  Scope : Scope
  Sum2 : Sum
  Switch : Switch  Threshold=1
  compute_position_errors : MATLAB Function  TreatAsAtomicUnit=on
  compute_velocity_error : MATLAB Function  TreatAsAtomicUnit=on
  Y : Outport
  wires:
  references/1 -> compute_position_errors/2(ref)
  compute_position_errors/1(err_pos) -> K_p_y_trans/1  "err_vect"
  K_p_y_trans/1 -> compute_velocity_error/2(v_des)
  "estimated measures "/1 -> compute_velocity_error/3(est_meas), compute_position_errors/3(est_state)
  compute_velocity_error/1(err_vel) -> K_i_sway_trans/1, K_p_sway_trans/1  "err_vel"
  Discrete-Time Integrator/1 -> Scope/1, Sum2/2
  K_i_sway_trans/1 -> Discrete-Time Integrator/1
  Sum2/1 -> Y/1
  K_p_sway_trans/1 -> Sum2/1
  Switch/1 -> Discrete-Time Integrator/2
  enable/1 -> Switch/2, compute_velocity_error/1(enable), compute_position_errors/1(enable)
  Constant1/1 -> Switch/3
  Constant/1 -> Switch/1

== system mixTest123/controller/transect controller/yaw_controller/Yaw PID controller ==
  enable : Inport
  references : Inport  Port=2
  "estimated measures " : Inport  Port=3
  Constant : Constant
  Constant1 : Constant  Value=0
  Discrete-Time Integrator : DiscreteIntegrator  ExternalReset=falling  SampleTime=0.1  ICPrevOutput=DiscIntNeverNeededParam  ICPrevScaledInput=DiscIntNeverNeededParam
  K_i_yaw_trans : Gain  Gain=K_i_yaw_trans
  K_p_psi_trans : Gain  Gain=K_p_psi_trans
  K_p_yaw_trans : Gain  Gain=K_p_yaw_trans
  Sum2 : Sum
  Switch : Switch  Threshold=1
  compute_orientation_errors : MATLAB Function  TreatAsAtomicUnit=on
  compute_velocity_error : MATLAB Function  TreatAsAtomicUnit=on
  N : Outport
  wires:
  references/1 -> compute_orientation_errors/2(ref)
  "estimated measures "/1 -> compute_velocity_error/3(est_meas), compute_orientation_errors/3(est_state)
  compute_orientation_errors/1(err_orient) -> K_p_psi_trans/1  "err_orient"
  K_p_psi_trans/1 -> compute_velocity_error/2(v_des)
  Sum2/1 -> N/1
  Discrete-Time Integrator/1 -> Sum2/2
  K_p_yaw_trans/1 -> Sum2/1
  K_i_yaw_trans/1 -> Discrete-Time Integrator/1
  compute_velocity_error/1(err_vel) -> K_i_yaw_trans/1, K_p_yaw_trans/1  "err_vel"
  Switch/1 -> Discrete-Time Integrator/2
  enable/1 -> Switch/2, compute_velocity_error/1(enable), compute_orientation_errors/1(enable)
  Constant1/1 -> Switch/3
  Constant/1 -> Switch/1

== system mixTest123/controller/turning controller/heave_controller/Heave PID controller ==
  enable : Inport
  references : Inport  Port=2
  "estimated measures " : Inport  Port=3
  Constant : Constant  Value=galleggiamento
  Constant1 : Constant
  Constant2 : Constant  Value=0
  Discrete-Time Integrator : DiscreteIntegrator  ExternalReset=falling  InitialConditionSource=external  SampleTime=0.1  ICPrevOutput=DiscIntNeverNeededParam  ICPrevScaledInput=DiscIntNeverNeededParam
  K_i_heave_turn : Gain  Gain=K_i_heave_turn
  K_p_heave_turn : Gain  Gain=K_p_heave_turn
  K_p_z_turn : Gain  Gain=K_p_z_turn
  Sum2 : Sum
  Switch : Switch  Threshold=1
  compute_position_errors : MATLAB Function  TreatAsAtomicUnit=on
  compute_velocity_error : MATLAB Function  TreatAsAtomicUnit=on
  Z : Outport
  wires:
  "estimated measures "/1 -> compute_velocity_error/3(est_meas), compute_position_errors/3(est_state)
  K_p_z_turn/1 -> compute_velocity_error/2(v_des)
  compute_position_errors/1(err_pos) -> K_p_z_turn/1  "err_vect"
  references/1 -> compute_position_errors/2(ref)
  K_p_heave_turn/1 -> Sum2/1
  K_i_heave_turn/1 -> Discrete-Time Integrator/1
  Discrete-Time Integrator/1 -> Sum2/2
  Sum2/1 -> Z/1
  compute_velocity_error/1(err_vel) -> K_i_heave_turn/1, K_p_heave_turn/1  "err_vel"
  Constant/1 -> Discrete-Time Integrator/3
  Switch/1 -> Discrete-Time Integrator/2
  enable/1 -> Switch/2, compute_velocity_error/1(enable), compute_position_errors/1(enable)
  Constant2/1 -> Switch/3
  Constant1/1 -> Switch/1

== system mixTest123/controller/turning controller/pitch_controller/Pitch PID controller ==
  enable : Inport
  references : Inport  Port=2
  "estimated measures " : Inport  Port=3
  Constant : Constant
  Constant1 : Constant  Value=0
  Discrete-Time Integrator : DiscreteIntegrator  ExternalReset=falling  SampleTime=0.1  ICPrevOutput=DiscIntNeverNeededParam  ICPrevScaledInput=DiscIntNeverNeededParam
  K_i_pitch_turn : Gain  Gain=K_i_pitch_turn
  K_p_pitch_turn : Gain  Gain=K_p_pitch_turn
  K_p_th_turn : Gain  Gain=K_p_th_turn
  Sum2 : Sum
  Switch : Switch  Threshold=1
  compute_orientation_errors : MATLAB Function  TreatAsAtomicUnit=on
  compute_velocity_error : MATLAB Function  TreatAsAtomicUnit=on
  M : Outport
  wires:
  references/1 -> compute_orientation_errors/2(ref)
  K_p_th_turn/1 -> compute_velocity_error/2(v_des)
  "estimated measures "/1 -> compute_velocity_error/3(est_meas), compute_orientation_errors/3(est_state)
  compute_orientation_errors/1(err_orient) -> K_p_th_turn/1  "err_orient"
  Sum2/1 -> M/1
  compute_velocity_error/1(err_vel) -> K_i_pitch_turn/1, K_p_pitch_turn/1  "err_vel"
  Discrete-Time Integrator/1 -> Sum2/2
  K_p_pitch_turn/1 -> Sum2/1
  K_i_pitch_turn/1 -> Discrete-Time Integrator/1
  Switch/1 -> Discrete-Time Integrator/2
  enable/1 -> Switch/2, compute_velocity_error/1(enable), compute_orientation_errors/1(enable)
  Constant1/1 -> Switch/3
  Constant/1 -> Switch/1

== system mixTest123/controller/turning controller/roll_controller/Roll PID controller ==
  enable : Inport
  references : Inport  Port=2
  "estimated measures " : Inport  Port=3
  Constant : Constant
  Constant1 : Constant  Value=0
  Discrete-Time Integrator : DiscreteIntegrator  ExternalReset=falling  SampleTime=0.1  ICPrevOutput=DiscIntNeverNeededParam  ICPrevScaledInput=DiscIntNeverNeededParam
  K_i_roll_turn : Gain  Gain=K_i_roll_turn
  K_p_phi_turn : Gain  Gain=K_p_phi_turn
  K_p_roll_turn : Gain  Gain=K_p_roll_turn
  Sum2 : Sum
  Switch : Switch  Threshold=1
  compute_orientation_errors : MATLAB Function  TreatAsAtomicUnit=on
  compute_velocity_error : MATLAB Function  TreatAsAtomicUnit=on
  K : Outport
  wires:
  "estimated measures "/1 -> compute_velocity_error/3(est_meas), compute_orientation_errors/3(est_state)
  K_p_phi_turn/1 -> compute_velocity_error/2(v_des)
  compute_orientation_errors/1(err_orient) -> K_p_phi_turn/1  "err_orient"
  references/1 -> compute_orientation_errors/2(ref)
  Sum2/1 -> K/1
  compute_velocity_error/1(err_vel) -> K_i_roll_turn/1, K_p_roll_turn/1  "err_vel"
  Discrete-Time Integrator/1 -> Sum2/2
  K_p_roll_turn/1 -> Sum2/1
  K_i_roll_turn/1 -> Discrete-Time Integrator/1
  Switch/1 -> Discrete-Time Integrator/2
  enable/1 -> Switch/2, compute_velocity_error/1(enable), compute_orientation_errors/1(enable)
  Constant1/1 -> Switch/3
  Constant/1 -> Switch/1

== system mixTest123/controller/turning controller/surge_controller/Surge PID controller ==
  enable : Inport
  ref : Inport  Port=2
  est_meas : Inport  Port=3
  " compute_velocity_error" : MATLAB Function  TreatAsAtomicUnit=on
  Constant : Constant
  Constant1 : Constant  Value=0
  Constant2 : Constant  Value=turning_surge
  Discrete-Time Integrator : DiscreteIntegrator  ExternalReset=falling  InitialConditionSource=external  SampleTime=0.1  ICPrevOutput=DiscIntNeverNeededParam  ICPrevScaledInput=DiscIntNeverNeededParam
  K_i_surge_turn : Gain  Gain=K_i_surge_turn
  K_p_surge_turn : Gain  Gain=K_p_surge_turn
  Scope : Scope
  Sum2 : Sum
  Switch : Switch  Threshold=1
  X : Outport
  wires:
  est_meas/1 -> " compute_velocity_error"/3(est_meas)
  ref/1 -> " compute_velocity_error"/2(ref)
  Sum2/1 -> Scope/1, X/1
  Discrete-Time Integrator/1 -> Sum2/2
  K_p_surge_turn/1 -> Sum2/1
  K_i_surge_turn/1 -> Discrete-Time Integrator/1
  " compute_velocity_error"/1(err_vel) -> K_i_surge_turn/1, K_p_surge_turn/1  "err_vel"
  Switch/1 -> Discrete-Time Integrator/2
  enable/1 -> Switch/2, " compute_velocity_error"/1(enable)
  Constant1/1 -> Switch/3
  Constant/1 -> Switch/1
  Constant2/1 -> Discrete-Time Integrator/3

== system mixTest123/controller/turning controller/sway_controller/Sway PID controller ==
  enable : Inport
  references : Inport  Port=2
  "estimated measures " : Inport  Port=3
  Constant : Constant
  Constant1 : Constant  Value=0
  Discrete-Time Integrator : DiscreteIntegrator  ExternalReset=falling  SampleTime=0.1  ICPrevOutput=DiscIntNeverNeededParam  ICPrevScaledInput=DiscIntNeverNeededParam
  K_i_sway_turn : Gain  Gain=K_i_sway_turn
  K_p_sway_turn : Gain  Gain=K_p_sway_turn
  K_p_y_turn : Gain  Gain=K_p_y_turn
  Scope : Scope
  Sum2 : Sum
  Switch : Switch  Threshold=1
  compute_position_errors : MATLAB Function  TreatAsAtomicUnit=on
  compute_velocity_error : MATLAB Function  TreatAsAtomicUnit=on
  Y : Outport
  wires:
  references/1 -> compute_position_errors/2(ref)
  compute_position_errors/1(err_pos) -> K_p_y_turn/1  "err_vect"
  K_p_y_turn/1 -> compute_velocity_error/2(v_des)
  "estimated measures "/1 -> compute_velocity_error/3(est_meas), compute_position_errors/3(est_state)
  K_p_sway_turn/1 -> Sum2/1
  K_i_sway_turn/1 -> Discrete-Time Integrator/1
  Discrete-Time Integrator/1 -> Scope/1, Sum2/2
  compute_velocity_error/1(err_vel) -> K_i_sway_turn/1, K_p_sway_turn/1  "err_vel"
  Sum2/1 -> Y/1
  Switch/1 -> Discrete-Time Integrator/2
  enable/1 -> Switch/2, compute_velocity_error/1(enable), compute_position_errors/1(enable)
  Constant1/1 -> Switch/3
  Constant/1 -> Switch/1
